simulink model "SIRmodel_Simulink"  (R2018a)
settings: Solver=VariableStepAuto  StartTime=0.0  StopTime=150  RelTol=1e-3
settings Model: Creator=Tech  LastModifiedBy=Tech

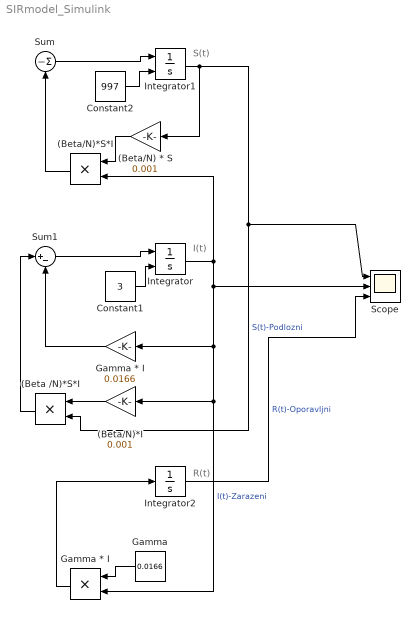
== system SIRmodel_Simulink ==
  note: S(t)
  note: I(t)
  note: R(t)
  " Gamma * I" : Product
  (Beta /N)*S*I : Product
  (Beta/N) * S : Gain  Gain=0.001
  (Beta/N)*I : Gain  Gain=0.001
  (Beta/N)*S*I : Product
  Constant1 : Constant  Value=3
  Constant2 : Constant  Value=997
  Gamma : Constant  Value=0.0166
  "Gamma * I " : Gain  Gain=0.0166
  Integrator : Integrator  InitialConditionSource=external
  Integrator1 : Integrator  InitialConditionSource=external  InitialCondition=1000
  Integrator2 : Integrator
  Scope : Scope  NumInputPorts=3
  Sum : Sum  Inputs=|-
  Sum1 : Sum  Inputs=|+-
  wires:
  Sum/1 -> Integrator1/1
  Sum1/1 -> Integrator/1
  Integrator/1 -> (Beta/N)*S*I/2, "Gamma * I "/1, (Beta/N)*I/1, " Gamma * I"/2, Scope/2  "I(t)-Zarazeni"
  "Gamma * I "/1 -> Sum1/2
  Integrator2/1 -> Scope/3  "R(t)-Oporavljni"
  " Gamma * I"/1 -> Integrator2/1
  (Beta/N) * S/1 -> (Beta/N)*S*I/1
  Integrator1/1 -> Scope/1, (Beta /N)*S*I/2, (Beta/N) * S/1  "S(t)-Podlozni"
  Gamma/1 -> " Gamma * I"/1
  Constant2/1 -> Integrator1/2
  Constant1/1 -> Integrator/2
  (Beta/N)*I/1 -> (Beta /N)*S*I/1
  (Beta /N)*S*I/1 -> Sum1/1
  (Beta/N)*S*I/1 -> Sum/1
